simulink model "No_1_Simulink"  (R2023b)
settings: Solver=VariableStepAuto  StartTime=0.0  StopTime=20  RelTol=1e-3
values from neighbouring files (symbols this model uses):
  G1_den = [1 0 0]    [No_1.m]    (also in No_2.m)
  G1_num = [1]    [No_1.m]    (also in No_2.m)
  G2_den = [1 1]    [No_1.m]    (also in No_2.m)
  G2_num = [1]    [No_1.m]    (also in No_2.m)
  G3_den = [1 0]    [No_1.m]    (also in No_2.m)
  G3_num = [1]    [No_1.m]    (also in No_2.m)
  H1_den = [1 0]    [No_1.m]    (also in No_2.m)
  H1_num = [1]    [No_1.m]    (also in No_2.m)
  H2_den = [1 -1]    [No_1.m]    (also in No_2.m)
  H2_num = [1]    [No_1.m]    (also in No_2.m)
  H3_den = [1 -2]    [No_1.m]    (also in No_2.m)
  H3_num = [1]    [No_1.m]    (also in No_2.m)
  TF_den = conv(TF4_den,TF6_den)    [No_1.m]
  TF_num = conv(TF4_num,TF6_num)    [No_1.m]
settings Model: Creator=ACER  LastModifiedBy=ACER

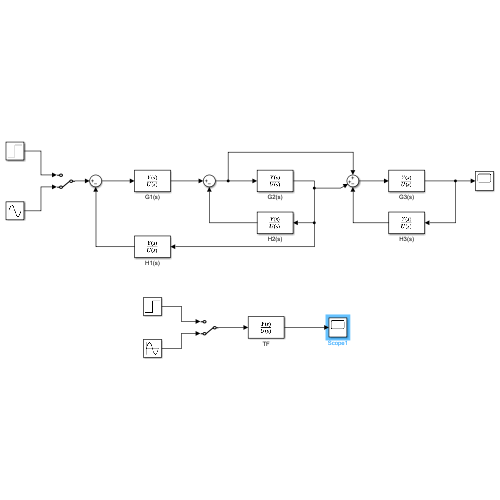
[thumbnail: Simulink's stored preview of the top-level diagram]
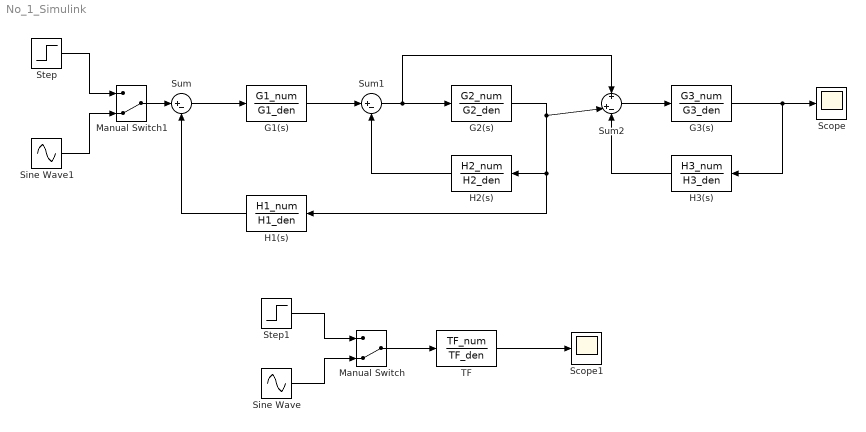
== system No_1_Simulink ==
  G1(s) : TransferFcn  Numerator=G1_num  Denominator=G1_den
  G2(s) : TransferFcn  Numerator=G2_num  Denominator=G2_den
  G3(s) : TransferFcn  Numerator=G3_num  Denominator=G3_den
  H1(s) : TransferFcn  Numerator=H1_num  Denominator=H1_den
  H2(s) : TransferFcn  Numerator=H2_num  Denominator=H2_den
  H3(s) : TransferFcn  Numerator=H3_num  Denominator=H3_den
  Manual Switch : ManualSwitch  CurrentSetting=0
  Manual Switch1 : ManualSwitch  CurrentSetting=0
  Scope : Scope
  Scope1 : Scope
  Sine Wave : Sin  SampleTime=0
  Sine Wave1 : Sin  SampleTime=0
  Step : Step  Time=0  SampleTime=0
  Step1 : Step  Time=0  SampleTime=0
  Sum : Sum  Inputs=|+-
  Sum1 : Sum  Inputs=|+-
  Sum2 : Sum  Inputs=+|+-
  TF : TransferFcn  Numerator=TF_num  Denominator=TF_den
  wires:
  Sum/1 -> G1(s)/1
  G1(s)/1 -> Sum1/1
  H2(s)/1 -> Sum1/2
  G2(s)/1 -> H1(s)/1, H2(s)/1, Sum2/2
  Sum1/1 -> Sum2/1, G2(s)/1
  H1(s)/1 -> Sum/2
  Sum2/1 -> G3(s)/1
  H3(s)/1 -> Sum2/3
  G3(s)/1 -> H3(s)/1, Scope/1
  TF/1 -> Scope1/1
  Manual Switch/1 -> TF/1
  Step1/1 -> Manual Switch/1
  Sine Wave/1 -> Manual Switch/2
  Manual Switch1/1 -> Sum/1
  Step/1 -> Manual Switch1/1
  Sine Wave1/1 -> Manual Switch1/2
